simulink model "Model_14Bus_Microgrid_paper_Latam"  (R2022b)
settings: Solver=VariableStepAuto  StartTime=0.0  StopTime=0.5  MaxStep=1e-2  RelTol=1e-3
InitFcn:
  | Set_parameters_R2018
StopFcn:
  | %Save_Data;
  | %Graphics_mod;
values from neighbouring files (symbols this model uses):
  Clink = Ceq*2    (= 0.217013888889)    [Set_parameters.m]
  dis1 = 0.15    [Set_parameters.m]
  dis10 = 6    [Set_parameters.m]
  dis11 = 3    [Set_parameters.m]
  dis12 = 6    [Set_parameters.m]
  dis13 = 3    [Set_parameters.m]
  dis14 = 2    [Set_parameters.m]
  dis2 = 0.2    [Set_parameters.m]
  dis3 = 0.15    [Set_parameters.m]
  dis4 = 0.4    [Set_parameters.m]
  dis5 = 0.4    [Set_parameters.m]
  dis6 = 0.4    [Set_parameters.m]
  dis7 = 0.1    [Set_parameters.m]
  dis8 = 2    [Set_parameters.m]
  dis9 = 6    [Set_parameters.m]
  Fc = 33 * Fnom    (= 1980)    [Set_parameters.m]
  Fnom = 60    [Set_parameters.m]
  Increment_MPPT = 0.01    [Set_parameters.m]
  Ki_Ireg = 20    [Set_parameters.m]
  Ki_VDCreg = 400    [Set_parameters.m]
  Kp_Ireg = 0.3    [Set_parameters.m]
  Kp_VDCreg = 2    [Set_parameters.m]
  LimitL_Ireg = -1.5    [Set_parameters.m]
  LimitL_VDCreg = -1.5    [Set_parameters.m]
  Limits_MPPT = [ 583 357 ]    [Set_parameters.m]
  LimitU_Ireg = 1.5    [Set_parameters.m]
  LimitU_VDCreg = 1.5    [Set_parameters.m]
  P_Load_2 = S_Load_2* PF_Load_2    (= 36000)    [Set_parameters.m]
  P_Load_3 = S_Load_3* PF_Load_3    (= 25500)    [Set_parameters.m]
  Pnom = 1e6    (= 1000000)    [Set_parameters.m]
  Pnom_T1 = 1.5e6    (= 1500000)    [Set_parameters.m]
  Pnom_T2 = 1.5e6    (= 1500000)    [Set_parameters.m]
  Pnom_T3 = 4e6    (= 4000000)    [Set_parameters.m]
  Pnom_xfo = Pnom    (= 1000000)    [Set_parameters.m]
  Ql_Load_2 = S_Load_2 * sin(acos(PF_Load_2))    [Set_parameters.m]
  Ql_Load_3 = S_Load_3 * sin(acos(PF_Load_3))    [Set_parameters.m]
  R_Load_9 = (Vnom_prim * 1.35)^2 / P_Load_9    (= 1084.6153125)    [Set_parameters.m]
  R_Load_DC = Vnom_DC^2/ P_Load_DC    (= 45)    [Set_parameters.m]
  Rl = 0.394    [Set_parameters.m]
  Rls = 0.198    [Set_parameters.m]
  Ts = Ts_Power    (= 5.05050505051e-06)    [Set_parameters.m]
  Ts_Control = 10*Ts_Power    (= 5.05050505051e-05)    [Set_parameters.m]
  Ts_Power = 1/(33*Fnom)/100    (= 5.05050505051e-06)    [Set_parameters.m]
  V1_LL_T3 = 69e3    (= 69000)    [Set_parameters.m]
  Vf = 0    [Set_parameters.m]
  Vfd = 0    [Set_parameters.m]
  Vnom_dc = 480    [Set_parameters.m]
  Vnom_Diesel = 2.4e3    (= 2400)    [Set_parameters.m]
  Vnom_prim = 13.8e3    (= 13800)    [Set_parameters.m]
  Vnom_sec = 220    [Set_parameters.m]
  Vnom_ter_AC_DC = 150    [Set_parameters.m]
  Xl = 0.1168    [Set_parameters.m]
  Xls = 0.1089    [Set_parameters.m]
undefined symbols (not defined in the file or in its folder): D1, Delta, DiscIntNeverNeededParam, Hydride, Ion, level, Lithium, max_min, Metal, Nickel, RL, RLff, sigbuilder_block
libraries: spsRMSLib x73, powerlib_extras x53, spsCurrentMeasurementLib x47, spsTHDLib x26, spsThreePhaseVIMeasurementLib x25, spsVoltageMeasurementLib x23, spsSeriesRLCBranchLib x21, spsThreePhaseSeriesRLCBranchLib x21, spsIGBTDiodeLib x15, spsThreePhaseBreakerLib x14, spsPowerLib x14, spsThreePhaseTransformerTwoWindingsLib x12
(part 2 of 10)

== system Model_14Bus_Microgrid_paper_Latam/BESS ==
  note: B1 + -
  note: + - B3
  note: + - B2
  note: DC Bus
  note: AC Bus
  note: ---------------
  note: -----------------
  "BESS " : Subsystem
      mask Display: image('/Users/christian/Documents/MATLAB/doctorado/4 conectada a la red con generador diesel, con generacion renovanble (fv)-con almacenamiento varios scope/Icons/Battery Energy Storage System (BESS).png'); % Use "Edit Image" on toolstrip to change.
  "Breaker BESS " : spsThreePhaseBreakerLib/Three-Phase Breaker  InitialState=closed  SwitchA=on  SwitchB=on  SwitchC=on  SwitchTimes="[4/60  10/60]"  External=on  BreakerResistance=0.001  SnubberResistance=1e6  SnubberCapacitance=inf  Measurements=None
  On/off Bess : Constant
  TB 900 V / 220 V 55 kVA : spsThreePhaseTransformerTwoWindingsLib/Three-Phase Transformer (Two Windings)  Winding1Connection=Delta (D1)  Winding2Connection=Y  CoreType=Three single-phase transformers  SetSaturation=off  Hysteresis=off  DataFile='hysteresis'  SetInitialFlux=off  Measurements=None  UNITS=pu  NominalPower=[ 55e3 , Fnom ]  Winding1=[ 900 , 0.0015 , 0.03]  Winding2=[ Vnom_sec , 0.0015 , 0.03 ]  Rm=200  Lm=200  L0=0.5  Saturation="[ 0,0  ;  0.005,1.2  ;  1.0,1.4 ]"  InitialFluxes=[ 0.8 , -0.8 , 0.7 ]  BreakLoop=off  DiscreteSolver=Trapezoidal iterative  DataType=off  TransfoNumber=0
  convertidor bidireccional AC/DC : Subsystem
      mask Display: image('/Users/christian/Documents/MATLAB/doctorado/4 conectada a la red con generador diesel, con generacion renovanble (fv)-con almacenamiento varios scope/Icons/Bi-directional converter.png'); % Use "Edit Image" on toolstrip to change.
  a : PMIOPort  Side=Right
  b : PMIOPort  Port=2  Side=Right
  c : PMIOPort  Port=3  Side=Right
  wires:
  On/off Bess/1 -> "Breaker BESS "/1
  connections:
  a/RConn1 -- "Breaker BESS "/RConn1
  TB 900 V / 220 V 55 kVA/LConn1 -- convertidor bidireccional AC/DC/LConn3
  TB 900 V / 220 V 55 kVA/RConn3 -- "Breaker BESS "/LConn3
  "BESS "/LConn5 -- convertidor bidireccional AC/DC/RConn2
  "Breaker BESS "/RConn3 -- c/RConn1
  "BESS "/LConn6 -- convertidor bidireccional AC/DC/RConn1
  TB 900 V / 220 V 55 kVA/LConn2 -- convertidor bidireccional AC/DC/LConn2
  TB 900 V / 220 V 55 kVA/LConn3 -- convertidor bidireccional AC/DC/LConn1
  "BESS "/LConn2 -- convertidor bidireccional AC/DC/RConn5
  "BESS "/LConn4 -- convertidor bidireccional AC/DC/RConn3
  TB 900 V / 220 V 55 kVA/RConn2 -- "Breaker BESS "/LConn2
  b/RConn1 -- "Breaker BESS "/RConn2
  TB 900 V / 220 V 55 kVA/RConn1 -- "Breaker BESS "/LConn1
  "BESS "/LConn1 -- convertidor bidireccional AC/DC/RConn6
  "BESS "/LConn3 -- convertidor bidireccional AC/DC/RConn4

== system Model_14Bus_Microgrid_paper_Latam/BESS2 ==
  note: ---------------------------------------------------------------------------
  Breaker : spsBreakerLib/Breaker  InitialState=1  SwitchingTimes="[1/60  5/60]"  External=on  BreakerResistance=0.01  SnubberResistance=1e6  SnubberCapacitance=inf  Measurements=None  MoreParameters=on  NoBreakLoop=off
  Breaker1 : spsBreakerLib/Breaker  InitialState=1  SwitchingTimes="[1/60  5/60]"  External=on  BreakerResistance=0.01  SnubberResistance=1e6  SnubberCapacitance=inf  Measurements=None  MoreParameters=on  NoBreakLoop=off
  Current Measurement1 : spsCurrentMeasurementLib/Current Measurement  PhasorSimulation=off  OutputType=Complex  PSBequivalent=0
  On/off 1 : Constant
  Subsystem2 : Subsystem
  1 : PMIOPort  Side=Left
  2 : PMIOPort  Port=2  Side=Left
  3 : PMIOPort  Port=3  Side=Right
  4 : PMIOPort  Port=4  Side=Right
  tag scope: I_BusDC=global
  wires:
  Current Measurement1/1 -> [I_BusDC]
  On/off 1/1 -> Breaker1/1, Breaker/1
  connections:
  1/RConn1 -- Breaker1/RConn1
  2/RConn1 -- Breaker/RConn1
  Subsystem2/RConn2 -- Breaker1/LConn1 -- 3/RConn1
  Current Measurement1/LConn1 -- Subsystem2/RConn1 -- 4/RConn1
  Current Measurement1/RConn1 -- Breaker/LConn1

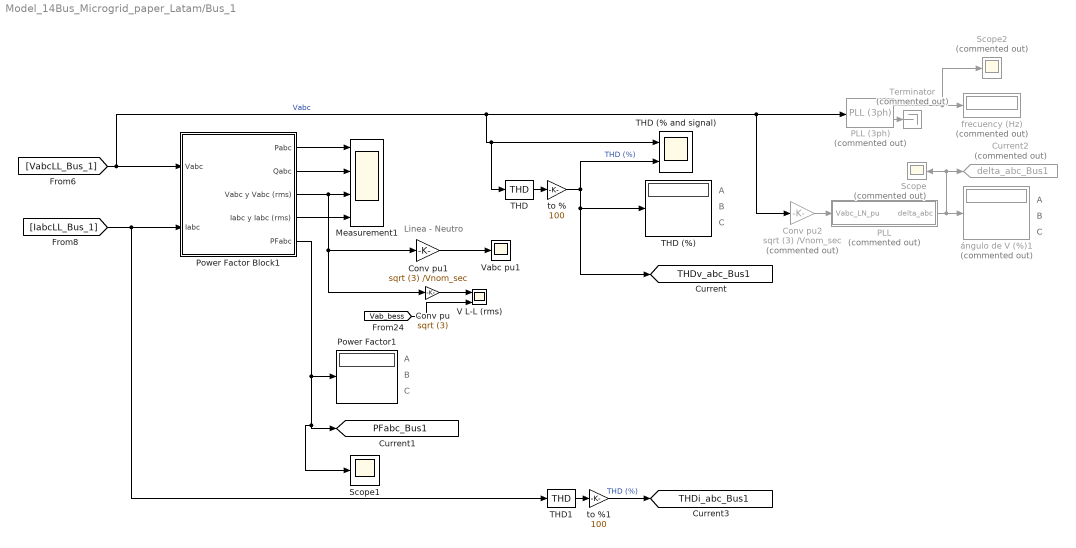
== system Model_14Bus_Microgrid_paper_Latam/Bus_1 ==
  note: C
  note: B
  note: A
  note: C
  note: Linea - Neutro
  note: B
  note: A
  note: A
  note: C
  note: B
  Conv pu : Gain  Gain=sqrt (3)  SaturateOnIntegerOverflow=on  OutDataTypeStr=Inherit: Same as input  ParamDataTypeStr=Inherit: Same as input
  Conv pu1 : Gain  Gain=sqrt (3) /Vnom_sec  SaturateOnIntegerOverflow=on  OutDataTypeStr=Inherit: Same as input  ParamDataTypeStr=Inherit: Same as input
  Conv pu2 : Gain  Commented=on  Gain=sqrt (3) /Vnom_sec  SaturateOnIntegerOverflow=on  OutDataTypeStr=Inherit: Same as input  ParamDataTypeStr=Inherit: Same as input
  Current2 : Goto  Commented=on  GotoTag=delta_abc_Bus1  TagVisibility=global
  Measurement1 : Scope  NumInputPorts=4
  PLL : Subsystem  Commented=on
  PLL (3ph) : spsPLL3phLib/PLL (3ph)  Commented=on  Fmin=45  Par_Init=[0, 60]  ParK=[180, 3200, 1]  TcD=1e-4  MaxRateChangeFreq=12  FilterCutOffFreq=25  Ts=0  AGC=on
  Power Factor Block1 : Subsystem  mask(Power Factor Block){Freq=Fnom, Vinit=[0, 0], Iinit=[0, 0], Ts=0}
      mask prompts: Freq "Fundamental frequency (Hz):"; Vinit "Voltage initial input [ Mag, Phase (degrees) ]:"; Iinit "Current initial input [ Mag, Phase (degrees) ]:"; Ts "Sample time:"
      mask help:
      | Power Factor Block developed by Dr Rodney Tan
      | Version 1.01 (Aug 2016)
      |
      | Compute power factor and phase angle of AC circuit voltage-current pair at fundamental frequency.
      |
      | The computation is based on Power block and Complex number function block.
      |
      | For the first cycle of simulation, the outputs are held constant to the powers computed for the Voltage initial input and Current initial input parameters.
      mask Help:
      | <b>Fundamental Frequency (Hz)</b>
      | Specify the measurement fundamental frequency, in hertz, of the input signal.
      | 
      | <b>Voltage initial input [ Mag, Phase (degrees) ]</b>
      | Specify the voltage initial magnitude and phase to set a constant output for the first cycle of simulation.
      | 
      | <b>Current initial input [ Mag, Phase (degrees) ]</b>
      | Specify the current initial magnitude and phase to set a constant output for the first cycle of simulation.
      | 
      | <b>Sample Time</b>
      | Specify the sample time of the block, in seconds. Set to 0 to implement a continuous block.
      mask TypeOptions Freq: Power/Freq
      mask TypeOptions Vinit: Power/Vinit
      mask TypeOptions Iinit: Power/Iinit
      mask TypeOptions Ts: Power/Ts
  Power Factor1 : Display
  Scope : Scope  Commented=on
  Scope1 : Scope
  Scope2 : Scope  Commented=on
  THD : spsTHDLib/THD  Freq=60  Ts=Ts_Power
  THD (% and signal) : Scope  NumInputPorts=2
  THD (%) : Display
      settings: Format=bank
  THD1 : spsTHDLib/THD  Freq=60  Ts=Ts_Power
  Terminator : Terminator  Commented=on
  V L-L (rms) : Scope  NumInputPorts=2
  Vabc pu1 : Scope
  frecuency (Hz) : Display  Commented=on
  to % : Gain  Gain=100  SampleTime=Ts_Power
  to %1 : Gain  Gain=100  SampleTime=Ts_Power
  ángulo de V (%)1 : Display  Commented=on
      settings: Format=bank
  tag scope: PFabc_Bus1=global, THDi_abc_Bus1=global, THDv_abc_Bus1=global
  wires:
  THD/1 -> to %/1
  to %/1 -> [THDv_abc_Bus1], THD (%)/1, THD (% and signal)/2  "THD (%)"
  Power Factor Block1/4(Iabc y Iabc (rms)) -> Measurement1/4
  Power Factor Block1/1(Pabc) -> Measurement1/1
  Conv pu1/1 -> Vabc pu1/1
  Power Factor Block1/5("PFabc ") -> Power Factor1/1, Scope1/1, [PFabc_Bus1]
  Power Factor Block1/2(Qabc) -> Measurement1/2
  Power Factor Block1/3(Vabc y Vabc (rms)) -> Conv pu/1, Conv pu1/1, Measurement1/3
  [IabcLL_Bus_1] -> THD1/1, Power Factor Block1/2(Iabc)
  Conv pu/1 -> V L-L (rms)/1
  [Vab_bess] -> V L-L (rms)/2
  PLL/1(delta_abc) -> Current2/1, Scope/1, ángulo de V (%)1/1
  Conv pu2/1 -> PLL/1(Vabc_LN_pu)
  PLL (3ph)/2 -> Terminator/1
  [VabcLL_Bus_1] -> Power Factor Block1/1(Vabc), PLL (3ph)/1, Conv pu2/1, THD/1, THD (% and signal)/1  "Vabc"
  PLL (3ph)/1 -> Scope2/1, frecuency (Hz)/1
  THD1/1 -> to %1/1
  to %1/1 -> [THDi_abc_Bus1]  "THD (%)"

== system Model_14Bus_Microgrid_paper_Latam/Bus_14  ==
  note: C
  note: B
  note: A
  note: C
  note: Linea - Neutro
  note: B
  note: A
  note: A
  note: B
  Conv pu1 : Gain  Gain=sqrt (3) /Vnom_prim  SaturateOnIntegerOverflow=on  OutDataTypeStr=Inherit: Same as input  ParamDataTypeStr=Inherit: Same as input
  Conv pu2 : Gain  Commented=on  Gain=sqrt (3) /Vnom_prim  SaturateOnIntegerOverflow=on  OutDataTypeStr=Inherit: Same as input  ParamDataTypeStr=Inherit: Same as input
  Current2 : Goto  Commented=on  GotoTag=delta_abc_Bus14  TagVisibility=global
  Gain : Gain  Gain=-1
  Measurement1 : Scope  NumInputPorts=4
  PLL : Subsystem  Commented=on
  Power Factor Block1 : Subsystem  mask(Power Factor Block){Freq=Fnom, Vinit=[0, 0], Iinit=[0, 0], Ts=0}
      mask prompts: Freq "Fundamental frequency (Hz):"; Vinit "Voltage initial input [ Mag, Phase (degrees) ]:"; Iinit "Current initial input [ Mag, Phase (degrees) ]:"; Ts "Sample time:"
      mask help:
      | Power Factor Block developed by Dr Rodney Tan
      | Version 1.01 (Aug 2016)
      |
      | Compute power factor and phase angle of AC circuit voltage-current pair at fundamental frequency.
      |
      | The computation is based on Power block and Complex number function block.
      |
      | For the first cycle of simulation, the outputs are held constant to the powers computed for the Voltage initial input and Current initial input parameters.
      mask Help:
      | <b>Fundamental Frequency (Hz)</b>
      | Specify the measurement fundamental frequency, in hertz, of the input signal.
      | 
      | <b>Voltage initial input [ Mag, Phase (degrees) ]</b>
      | Specify the voltage initial magnitude and phase to set a constant output for the first cycle of simulation.
      | 
      | <b>Current initial input [ Mag, Phase (degrees) ]</b>
      | Specify the current initial magnitude and phase to set a constant output for the first cycle of simulation.
      | 
      | <b>Sample Time</b>
      | Specify the sample time of the block, in seconds. Set to 0 to implement a continuous block.
      mask TypeOptions Freq: Power/Freq
      mask TypeOptions Vinit: Power/Vinit
      mask TypeOptions Iinit: Power/Iinit
      mask TypeOptions Ts: Power/Ts
  Power Factor1 : Display
  Scope : Scope  Commented=on
  THD : spsTHDLib/THD  Freq=60  Ts=Ts_Power
  THD (% and signal) : Scope  NumInputPorts=2
  THD (%) : Display
      settings: Format=bank
  THD1 : spsTHDLib/THD  Freq=60  Ts=Ts_Power
  Vabc pu1 : Scope
  to % : Gain  Gain=100  SampleTime=Ts_Power
  to %1 : Gain  Gain=100  SampleTime=Ts_Power
  ángulo de V (%)1 : Display  Commented=on
      settings: Format=bank
  tag scope: PFabc_Bus14=global, THDi_abc_Bus14=global, THDv_abc_Bus14=global
  wires:
  [IabcLL_Bus_14] -> THD1/1, Power Factor Block1/2(Iabc)
  THD/1 -> to %/1
  Power Factor Block1/4(Iabc y Iabc (rms)) -> Measurement1/4
  Power Factor Block1/1(Pabc) -> Measurement1/1
  Conv pu1/1 -> Vabc pu1/1
  Power Factor Block1/2(Qabc) -> Measurement1/2
  Power Factor Block1/3(Vabc y Vabc (rms)) -> Conv pu1/1, Measurement1/3
  to %/1 -> [THDv_abc_Bus14], THD (%)/1, THD (% and signal)/2  "THD (%)"
  Power Factor Block1/5("PFabc ") -> Gain/1
  PLL/1(delta_abc) -> Current2/1, Scope/1, ángulo de V (%)1/1
  [VabcLL_Bus_14] -> Power Factor Block1/1(Vabc), Conv pu2/1, THD/1, THD (% and signal)/1  "Signal Vabc"
  Conv pu2/1 -> PLL/1(Vabc_LN_pu)
  Gain/1 -> [PFabc_Bus14], Power Factor1/1
  THD1/1 -> to %1/1
  to %1/1 -> [THDi_abc_Bus14]  "THD (%)"

== system Model_14Bus_Microgrid_paper_Latam/Bus_2 ==
  note: C
  note: B
  note: A
  note: A
  note: B
  note: Linea - Neutro
  note: C
  note: A
  note: B
  note: C
  Conv pu1 : Gain  Gain=sqrt (3) /Vnom_sec  SaturateOnIntegerOverflow=on  OutDataTypeStr=Inherit: Same as input  ParamDataTypeStr=Inherit: Same as input
  Conv pu2 : Gain  Commented=on  Gain=sqrt (3) /Vnom_sec  SaturateOnIntegerOverflow=on  OutDataTypeStr=Inherit: Same as input  ParamDataTypeStr=Inherit: Same as input
  Current2 : Goto  Commented=on  GotoTag=delta_abc_Bus2  TagVisibility=global
  Measurement1 : Scope  NumInputPorts=4
  PLL : Subsystem  Commented=on
  PLL (3ph) : spsPLL3phLib/PLL (3ph)  Commented=on  Fmin=45  Par_Init=[0, 60]  ParK=[180, 3200, 1]  TcD=1e-4  MaxRateChangeFreq=12  FilterCutOffFreq=25  Ts=0  AGC=on
  Power Factor Block1 : Subsystem  mask(Power Factor Block){Freq=Fnom, Vinit=[0, 0], Iinit=[0, 0], Ts=0}
      mask prompts: Freq "Fundamental frequency (Hz):"; Vinit "Voltage initial input [ Mag, Phase (degrees) ]:"; Iinit "Current initial input [ Mag, Phase (degrees) ]:"; Ts "Sample time:"
      mask help:
      | Power Factor Block developed by Dr Rodney Tan
      | Version 1.01 (Aug 2016)
      |
      | Compute power factor and phase angle of AC circuit voltage-current pair at fundamental frequency.
      |
      | The computation is based on Power block and Complex number function block.
      |
      | For the first cycle of simulation, the outputs are held constant to the powers computed for the Voltage initial input and Current initial input parameters.
      mask Help:
      | <b>Fundamental Frequency (Hz)</b>
      | Specify the measurement fundamental frequency, in hertz, of the input signal.
      | 
      | <b>Voltage initial input [ Mag, Phase (degrees) ]</b>
      | Specify the voltage initial magnitude and phase to set a constant output for the first cycle of simulation.
      | 
      | <b>Current initial input [ Mag, Phase (degrees) ]</b>
      | Specify the current initial magnitude and phase to set a constant output for the first cycle of simulation.
      | 
      | <b>Sample Time</b>
      | Specify the sample time of the block, in seconds. Set to 0 to implement a continuous block.
      mask TypeOptions Freq: Power/Freq
      mask TypeOptions Vinit: Power/Vinit
      mask TypeOptions Iinit: Power/Iinit
      mask TypeOptions Ts: Power/Ts
  Power Factor1 : Display
  Scope : Scope  Commented=on
  Scope2 : Scope  Commented=on
  THD : spsTHDLib/THD  Freq=60  Ts=Ts_Power
  THD (% and signal) : Scope  NumInputPorts=2
  THD (%) : Display
      settings: Format=bank
  THD1 : spsTHDLib/THD  Freq=60  Ts=Ts_Power
  Terminator : Terminator  Commented=on
  Vabc pu1 : Scope
  frecuency (Hz) : Display  Commented=on
  to % : Gain  Gain=100  SampleTime=Ts_Power
  to %1 : Gain  Gain=100  SampleTime=Ts_Power
  ángulo de V (%)1 : Display  Commented=on
      settings: Format=bank
  tag scope: PFabc_Bus2=global, THDi_abc_Bus2=global, THDv_abc_Bus2=global
  wires:
  [IabcLL_Bus_2] -> THD1/1, Power Factor Block1/2(Iabc)
  THD/1 -> to %/1
  Power Factor Block1/3(Vabc y Vabc (rms)) -> Conv pu1/1, Measurement1/3
  Power Factor Block1/4(Iabc y Iabc (rms)) -> Measurement1/4
  Conv pu1/1 -> Vabc pu1/1
  Power Factor Block1/2(Qabc) -> Measurement1/2
  Power Factor Block1/1(Pabc) -> Measurement1/1
  Power Factor Block1/5("PFabc ") -> [PFabc_Bus2], Power Factor1/1
  to %/1 -> [THDv_abc_Bus2], THD (%)/1, THD (% and signal)/2  "THD (%)"
  Conv pu2/1 -> PLL/1(Vabc_LN_pu)
  PLL/1(delta_abc) -> Current2/1, Scope/1, ángulo de V (%)1/1
  PLL (3ph)/2 -> Terminator/1
  [VabcLL_Bus_2] -> PLL (3ph)/1, Conv pu2/1, THD/1, THD (% and signal)/1, Power Factor Block1/1(Vabc)  "Vabc"
  PLL (3ph)/1 -> Scope2/1, frecuency (Hz)/1
  THD1/1 -> to %1/1
  to %1/1 -> [THDi_abc_Bus2]  "THD (%)"

== system Model_14Bus_Microgrid_paper_Latam/Bus_3 ==
  note: C
  note: B
  note: A
  note: C
  note: Linea - Neutro
  note: B
  note: A
  note: A
  note: B
  note: C
  Conv pu1 : Gain  Gain=sqrt (3) /Vnom_sec  SaturateOnIntegerOverflow=on  OutDataTypeStr=Inherit: Same as input  ParamDataTypeStr=Inherit: Same as input
  Conv pu2 : Gain  Commented=on  Gain=sqrt (3) /Vnom_sec  SaturateOnIntegerOverflow=on  OutDataTypeStr=Inherit: Same as input  ParamDataTypeStr=Inherit: Same as input
  Current2 : Goto  Commented=on  GotoTag=delta_abc_Bus3  TagVisibility=global
  Measurement1 : Scope  NumInputPorts=4
  PLL : Subsystem  Commented=on
  Power Factor Block1 : Subsystem  mask(Power Factor Block){Freq=Fnom, Vinit=[0, 0], Iinit=[0, 0], Ts=0}
      mask prompts: Freq "Fundamental frequency (Hz):"; Vinit "Voltage initial input [ Mag, Phase (degrees) ]:"; Iinit "Current initial input [ Mag, Phase (degrees) ]:"; Ts "Sample time:"
      mask help:
      | Power Factor Block developed by Dr Rodney Tan
      | Version 1.01 (Aug 2016)
      |
      | Compute power factor and phase angle of AC circuit voltage-current pair at fundamental frequency.
      |
      | The computation is based on Power block and Complex number function block.
      |
      | For the first cycle of simulation, the outputs are held constant to the powers computed for the Voltage initial input and Current initial input parameters.
      mask Help:
      | <b>Fundamental Frequency (Hz)</b>
      | Specify the measurement fundamental frequency, in hertz, of the input signal.
      | 
      | <b>Voltage initial input [ Mag, Phase (degrees) ]</b>
      | Specify the voltage initial magnitude and phase to set a constant output for the first cycle of simulation.
      | 
      | <b>Current initial input [ Mag, Phase (degrees) ]</b>
      | Specify the current initial magnitude and phase to set a constant output for the first cycle of simulation.
      | 
      | <b>Sample Time</b>
      | Specify the sample time of the block, in seconds. Set to 0 to implement a continuous block.
      mask TypeOptions Freq: Power/Freq
      mask TypeOptions Vinit: Power/Vinit
      mask TypeOptions Iinit: Power/Iinit
      mask TypeOptions Ts: Power/Ts
  Power Factor1 : Display
  Scope : Scope  Commented=on
  THD : spsTHDLib/THD  Freq=60  Ts=Ts_Power
  THD (% and signal) : Scope  NumInputPorts=2
  THD (%) : Display
      settings: Format=bank
  THD1 : spsTHDLib/THD  Freq=60  Ts=Ts_Power
  Vabc pu1 : Scope
  to % : Gain  Gain=100  SampleTime=Ts_Power
  to %1 : Gain  Gain=100  SampleTime=Ts_Power
  ángulo de V (%)1 : Display  Commented=on
      settings: Format=bank
  tag scope: PFabc_Bus3=global, THDi_abc_Bus3=global, THDv_abc_Bus3=global
  wires:
  [IabcLL_Bus_3] -> THD1/1, Power Factor Block1/2(Iabc)
  THD/1 -> to %/1
  Power Factor Block1/4(Iabc y Iabc (rms)) -> Measurement1/4
  Power Factor Block1/1(Pabc) -> Measurement1/1
  Conv pu1/1 -> Vabc pu1/1
  Power Factor Block1/2(Qabc) -> Measurement1/2
  Power Factor Block1/3(Vabc y Vabc (rms)) -> Conv pu1/1, Measurement1/3
  Power Factor Block1/5("PFabc ") -> [PFabc_Bus3], Power Factor1/1
  to %/1 -> [THDv_abc_Bus3], THD (%)/1, THD (% and signal)/2  "THD (%)"
  Conv pu2/1 -> PLL/1(Vabc_LN_pu)
  PLL/1(delta_abc) -> Current2/1, Scope/1, ángulo de V (%)1/1
  [VabcLL_Bus_3] -> Conv pu2/1, THD/1, THD (% and signal)/1, Power Factor Block1/1(Vabc)  "Signal Vabc"
  THD1/1 -> to %1/1
  to %1/1 -> [THDi_abc_Bus3]  "THD (%)"

== system Model_14Bus_Microgrid_paper_Latam/Bus_4 ==
  note: C
  note: B
  note: A
  note: C
  note: Linea - Neutro
  note: B
  note: A
  note: A
  note: B
  note: C
  Conv pu1 : Gain  Gain=sqrt (3) /Vnom_sec  SaturateOnIntegerOverflow=on  OutDataTypeStr=Inherit: Same as input  ParamDataTypeStr=Inherit: Same as input
  Conv pu2 : Gain  Commented=on  Gain=sqrt (3) /Vnom_sec  SaturateOnIntegerOverflow=on  OutDataTypeStr=Inherit: Same as input  ParamDataTypeStr=Inherit: Same as input
  Current2 : Goto  Commented=on  GotoTag=delta_abc_Bus4  TagVisibility=global
  Measurement1 : Scope  NumInputPorts=4
  PLL : Subsystem  Commented=on
  Power Factor Block1 : Subsystem  mask(Power Factor Block){Freq=Fnom, Vinit=[0, 0], Iinit=[0, 0], Ts=0}
      mask prompts: Freq "Fundamental frequency (Hz):"; Vinit "Voltage initial input [ Mag, Phase (degrees) ]:"; Iinit "Current initial input [ Mag, Phase (degrees) ]:"; Ts "Sample time:"
      mask help:
      | Power Factor Block developed by Dr Rodney Tan
      | Version 1.01 (Aug 2016)
      |
      | Compute power factor and phase angle of AC circuit voltage-current pair at fundamental frequency.
      |
      | The computation is based on Power block and Complex number function block.
      |
      | For the first cycle of simulation, the outputs are held constant to the powers computed for the Voltage initial input and Current initial input parameters.
      mask Help:
      | <b>Fundamental Frequency (Hz)</b>
      | Specify the measurement fundamental frequency, in hertz, of the input signal.
      | 
      | <b>Voltage initial input [ Mag, Phase (degrees) ]</b>
      | Specify the voltage initial magnitude and phase to set a constant output for the first cycle of simulation.
      | 
      | <b>Current initial input [ Mag, Phase (degrees) ]</b>
      | Specify the current initial magnitude and phase to set a constant output for the first cycle of simulation.
      | 
      | <b>Sample Time</b>
      | Specify the sample time of the block, in seconds. Set to 0 to implement a continuous block.
      mask TypeOptions Freq: Power/Freq
      mask TypeOptions Vinit: Power/Vinit
      mask TypeOptions Iinit: Power/Iinit
      mask TypeOptions Ts: Power/Ts
  Power Factor1 : Display
  Scope : Scope  Commented=on
  THD : spsTHDLib/THD  Freq=60  Ts=Ts_Power
  THD (% and signal) : Scope  NumInputPorts=2
  THD (%) : Display
      settings: Format=bank
  THD1 : spsTHDLib/THD  Freq=60  Ts=Ts_Power
  Vabc pu1 : Scope
  to % : Gain  Gain=100  SampleTime=Ts_Power
  to %1 : Gain  Gain=100  SampleTime=Ts_Power
  ángulo de V (%)1 : Display  Commented=on
      settings: Format=bank
  tag scope: PFabc_Bus4=global, THDi_abc_Bus4=global, THDv_abc_Bus4=global
  wires:
  [IabcLL_Bus_4] -> THD1/1, Power Factor Block1/2(Iabc)
  THD/1 -> to %/1
  Power Factor Block1/4(Iabc y Iabc (rms)) -> Measurement1/4
  Power Factor Block1/1(Pabc) -> Measurement1/1
  Conv pu1/1 -> Vabc pu1/1
  Power Factor Block1/2(Qabc) -> Measurement1/2
  Power Factor Block1/3(Vabc y Vabc (rms)) -> Conv pu1/1, Measurement1/3
  Power Factor Block1/5("PFabc ") -> [PFabc_Bus4], Power Factor1/1
  to %/1 -> [THDv_abc_Bus4], THD (%)/1, THD (% and signal)/2  "THD (%)"
  Conv pu2/1 -> PLL/1(Vabc_LN_pu)
  PLL/1(delta_abc) -> Current2/1, Scope/1, ángulo de V (%)1/1
  [VabcLL_Bus_4] -> Power Factor Block1/1(Vabc), Conv pu2/1, THD/1, THD (% and signal)/1  "Signal Vabc"
  THD1/1 -> to %1/1
  to %1/1 -> [THDi_abc_Bus4]  "THD (%)"

== system Model_14Bus_Microgrid_paper_Latam/Bus_5 ==
  note: C
  note: B
  note: A
  note: C
  note: Linea - Neutro
  note: B
  note: A
  note: A
  note: B
  note: C
  Conv pu1 : Gain  Gain=sqrt (3) /Vnom_sec  SaturateOnIntegerOverflow=on  OutDataTypeStr=Inherit: Same as input  ParamDataTypeStr=Inherit: Same as input
  Conv pu2 : Gain  Commented=on  Gain=sqrt (3) /Vnom_sec  SaturateOnIntegerOverflow=on  OutDataTypeStr=Inherit: Same as input  ParamDataTypeStr=Inherit: Same as input
  Current2 : Goto  Commented=on  GotoTag=delta_abc_Bus5  TagVisibility=global
  Measurement1 : Scope  NumInputPorts=4
  PLL : Subsystem  Commented=on
  Power Factor Block1 : Subsystem  mask(Power Factor Block){Freq=Fnom, Vinit=[0, 0], Iinit=[0, 0], Ts=0}
      mask prompts: Freq "Fundamental frequency (Hz):"; Vinit "Voltage initial input [ Mag, Phase (degrees) ]:"; Iinit "Current initial input [ Mag, Phase (degrees) ]:"; Ts "Sample time:"
      mask help:
      | Power Factor Block developed by Dr Rodney Tan
      | Version 1.01 (Aug 2016)
      |
      | Compute power factor and phase angle of AC circuit voltage-current pair at fundamental frequency.
      |
      | The computation is based on Power block and Complex number function block.
      |
      | For the first cycle of simulation, the outputs are held constant to the powers computed for the Voltage initial input and Current initial input parameters.
      mask Help:
      | <b>Fundamental Frequency (Hz)</b>
      | Specify the measurement fundamental frequency, in hertz, of the input signal.
      | 
      | <b>Voltage initial input [ Mag, Phase (degrees) ]</b>
      | Specify the voltage initial magnitude and phase to set a constant output for the first cycle of simulation.
      | 
      | <b>Current initial input [ Mag, Phase (degrees) ]</b>
      | Specify the current initial magnitude and phase to set a constant output for the first cycle of simulation.
      | 
      | <b>Sample Time</b>
      | Specify the sample time of the block, in seconds. Set to 0 to implement a continuous block.
      mask TypeOptions Freq: Power/Freq
      mask TypeOptions Vinit: Power/Vinit
      mask TypeOptions Iinit: Power/Iinit
      mask TypeOptions Ts: Power/Ts
  Power Factor1 : Display
  Scope : Scope  Commented=on
  THD : spsTHDLib/THD  Freq=60  Ts=Ts_Power
  THD (% and signal) : Scope  NumInputPorts=2
  THD (%) : Display
      settings: Format=bank
  THD1 : spsTHDLib/THD  Freq=60  Ts=Ts_Power
  Vabc pu1 : Scope
  to % : Gain  Gain=100  SampleTime=Ts_Power
  to %1 : Gain  Gain=100  SampleTime=Ts_Power
  ángulo de V (%)1 : Display  Commented=on
      settings: Format=bank
  tag scope: PFabc_Bus5=global, THDi_abc_Bus5=global, THDv_abc_Bus5=global
  wires:
  [IabcLL_Bus_5] -> THD1/1, Power Factor Block1/2(Iabc)
  THD/1 -> to %/1
  Power Factor Block1/4(Iabc y Iabc (rms)) -> Measurement1/4
  Power Factor Block1/1(Pabc) -> Measurement1/1
  Conv pu1/1 -> Vabc pu1/1
  Power Factor Block1/2(Qabc) -> Measurement1/2
  Power Factor Block1/3(Vabc y Vabc (rms)) -> Conv pu1/1, Measurement1/3
  Power Factor Block1/5("PFabc ") -> [PFabc_Bus5], Power Factor1/1
  to %/1 -> [THDv_abc_Bus5], THD (%)/1, THD (% and signal)/2  "THD (%)"
  Conv pu2/1 -> PLL/1(Vabc_LN_pu)
  PLL/1(delta_abc) -> Current2/1, Scope/1, ángulo de V (%)1/1
  [VabcLL_Bus_5] -> Power Factor Block1/1(Vabc), Conv pu2/1, THD/1, THD (% and signal)/1  "Signal Vabc"
  THD1/1 -> to %1/1
  to %1/1 -> [THDi_abc_Bus5]  "THD (%)"

== system Model_14Bus_Microgrid_paper_Latam/Bus_6 ==
  note: C
  note: B
  note: A
  note: C
  note: Linea - Neutro
  note: B
  note: A
  note: A
  note: B
  note: C
  Conv pu1 : Gain  Gain=sqrt (3) /Vnom_sec  SaturateOnIntegerOverflow=on  OutDataTypeStr=Inherit: Same as input  ParamDataTypeStr=Inherit: Same as input
  Conv pu2 : Gain  Commented=on  Gain=sqrt (3) /Vnom_sec  SaturateOnIntegerOverflow=on  OutDataTypeStr=Inherit: Same as input  ParamDataTypeStr=Inherit: Same as input
  Current2 : Goto  Commented=on  GotoTag=delta_abc_Bus4  TagVisibility=global
  Measurement1 : Scope  NumInputPorts=4
  PLL : Subsystem  Commented=on
  Power Factor Block1 : Subsystem  mask(Power Factor Block){Freq=Fnom, Vinit=[0, 0], Iinit=[0, 0], Ts=0}
      mask prompts: Freq "Fundamental frequency (Hz):"; Vinit "Voltage initial input [ Mag, Phase (degrees) ]:"; Iinit "Current initial input [ Mag, Phase (degrees) ]:"; Ts "Sample time:"
      mask help:
      | Power Factor Block developed by Dr Rodney Tan
      | Version 1.01 (Aug 2016)
      |
      | Compute power factor and phase angle of AC circuit voltage-current pair at fundamental frequency.
      |
      | The computation is based on Power block and Complex number function block.
      |
      | For the first cycle of simulation, the outputs are held constant to the powers computed for the Voltage initial input and Current initial input parameters.
      mask Help:
      | <b>Fundamental Frequency (Hz)</b>
      | Specify the measurement fundamental frequency, in hertz, of the input signal.
      | 
      | <b>Voltage initial input [ Mag, Phase (degrees) ]</b>
      | Specify the voltage initial magnitude and phase to set a constant output for the first cycle of simulation.
      | 
      | <b>Current initial input [ Mag, Phase (degrees) ]</b>
      | Specify the current initial magnitude and phase to set a constant output for the first cycle of simulation.
      | 
      | <b>Sample Time</b>
      | Specify the sample time of the block, in seconds. Set to 0 to implement a continuous block.
      mask TypeOptions Freq: Power/Freq
      mask TypeOptions Vinit: Power/Vinit
      mask TypeOptions Iinit: Power/Iinit
      mask TypeOptions Ts: Power/Ts
  Power Factor1 : Display
  Scope : Scope  Commented=on
  THD : spsTHDLib/THD  Freq=60  Ts=Ts_Power
  THD (% and signal) : Scope  NumInputPorts=2
  THD (%) : Display
      settings: Format=bank
  THD1 : spsTHDLib/THD  Freq=60  Ts=Ts_Power
  Vabc pu1 : Scope
  to % : Gain  Gain=100  SampleTime=Ts_Power
  to %1 : Gain  Gain=100  SampleTime=Ts_Power
  ángulo de V (%)1 : Display  Commented=on
      settings: Format=bank
  tag scope: PFabc_Bus4=global, THDi_abc_Bus4=global, THDv_abc_Bus4=global
  wires:
  [IabcLL_Bus_4] -> THD1/1, Power Factor Block1/2(Iabc)
  THD/1 -> to %/1
  Power Factor Block1/4(Iabc y Iabc (rms)) -> Measurement1/4
  Power Factor Block1/1(Pabc) -> Measurement1/1
  Conv pu1/1 -> Vabc pu1/1
  Power Factor Block1/2(Qabc) -> Measurement1/2
  Power Factor Block1/3(Vabc y Vabc (rms)) -> Conv pu1/1, Measurement1/3
  Power Factor Block1/5("PFabc ") -> [PFabc_Bus4], Power Factor1/1
  to %/1 -> [THDv_abc_Bus4], THD (%)/1, THD (% and signal)/2  "THD (%)"
  Conv pu2/1 -> PLL/1(Vabc_LN_pu)
  PLL/1(delta_abc) -> Current2/1, Scope/1, ángulo de V (%)1/1
  [VabcLL_Bus_4] -> Power Factor Block1/1(Vabc), Conv pu2/1, THD/1, THD (% and signal)/1  "Signal Vabc"
  THD1/1 -> to %1/1
  to %1/1 -> [THDi_abc_Bus4]  "THD (%)"

== system Model_14Bus_Microgrid_paper_Latam/Bus_6  ==
  note: C
  note: B
  note: A
  note: C
  note: Linea - Neutro
  note: B
  note: A
  note: A
  note: B
  Conv pu1 : Gain  Gain=sqrt (3) /Vnom_prim  SaturateOnIntegerOverflow=on  OutDataTypeStr=Inherit: Same as input  ParamDataTypeStr=Inherit: Same as input
  Conv pu2 : Gain  Commented=on  Gain=sqrt (3) /Vnom_prim  SaturateOnIntegerOverflow=on  OutDataTypeStr=Inherit: Same as input  ParamDataTypeStr=Inherit: Same as input
  Current2 : Goto  Commented=on  GotoTag=delta_abc_Bus6  TagVisibility=global
  Measurement1 : Scope  NumInputPorts=4
  PLL : Subsystem  Commented=on
  PLL (3ph) : spsPLL3phLib/PLL (3ph)  Commented=on  Fmin=45  Par_Init=[0, 60]  ParK=[180, 3200, 1]  TcD=1e-4  MaxRateChangeFreq=12  FilterCutOffFreq=25  Ts=0  AGC=on
  Power Factor Block1 : Subsystem  mask(Power Factor Block){Freq=Fnom, Vinit=[0, 0], Iinit=[0, 0], Ts=0}
      mask prompts: Freq "Fundamental frequency (Hz):"; Vinit "Voltage initial input [ Mag, Phase (degrees) ]:"; Iinit "Current initial input [ Mag, Phase (degrees) ]:"; Ts "Sample time:"
      mask help:
      | Power Factor Block developed by Dr Rodney Tan
      | Version 1.01 (Aug 2016)
      |
      | Compute power factor and phase angle of AC circuit voltage-current pair at fundamental frequency.
      |
      | The computation is based on Power block and Complex number function block.
      |
      | For the first cycle of simulation, the outputs are held constant to the powers computed for the Voltage initial input and Current initial input parameters.
      mask Help:
      | <b>Fundamental Frequency (Hz)</b>
      | Specify the measurement fundamental frequency, in hertz, of the input signal.
      | 
      | <b>Voltage initial input [ Mag, Phase (degrees) ]</b>
      | Specify the voltage initial magnitude and phase to set a constant output for the first cycle of simulation.
      | 
      | <b>Current initial input [ Mag, Phase (degrees) ]</b>
      | Specify the current initial magnitude and phase to set a constant output for the first cycle of simulation.
      | 
      | <b>Sample Time</b>
      | Specify the sample time of the block, in seconds. Set to 0 to implement a continuous block.
      mask TypeOptions Freq: Power/Freq
      mask TypeOptions Vinit: Power/Vinit
      mask TypeOptions Iinit: Power/Iinit
      mask TypeOptions Ts: Power/Ts
  Power Factor1 : Display
  Scope : Scope  Commented=on
  Scope2 : Scope  Commented=on
  THD : spsTHDLib/THD  Freq=60  Ts=Ts_Power
  THD (% and signal) : Scope  NumInputPorts=2
  THD (%) : Display
      settings: Format=bank
  THD1 : spsTHDLib/THD  Freq=60  Ts=Ts_Power
  Terminator : Terminator  Commented=on
  Vabc pu1 : Scope
  frecuency (Hz) : Display  Commented=on
  to % : Gain  Gain=100  SampleTime=Ts_Power
  to %1 : Gain  Gain=100  SampleTime=Ts_Power
  ángulo de V (%)1 : Display  Commented=on
      settings: Format=bank
  tag scope: PFabc_Bus6=global, THDi_abc_Bus6=global, THDv_abc_Bus6=global
  wires:
  [IabcLL_Bus_6] -> THD1/1, Power Factor Block1/2(Iabc)
  THD/1 -> to %/1
  Power Factor Block1/4(Iabc y Iabc (rms)) -> Measurement1/4
  Power Factor Block1/1(Pabc) -> Measurement1/1
  Conv pu1/1 -> Vabc pu1/1
  Power Factor Block1/2(Qabc) -> Measurement1/2
  Power Factor Block1/3(Vabc y Vabc (rms)) -> Conv pu1/1, Measurement1/3
  Power Factor Block1/5("PFabc ") -> [PFabc_Bus6], Power Factor1/1
  to %/1 -> [THDv_abc_Bus6], THD (%)/1, THD (% and signal)/2  "THD (%)"
  PLL/1(delta_abc) -> Current2/1, Scope/1, ángulo de V (%)1/1
  Conv pu2/1 -> PLL/1(Vabc_LN_pu)
  PLL (3ph)/2 -> Terminator/1
  [VabcLL_Bus_6] -> Power Factor Block1/1(Vabc), Conv pu2/1, PLL (3ph)/1, THD/1, THD (% and signal)/1  "Vabc"
  PLL (3ph)/1 -> Scope2/1, frecuency (Hz)/1
  THD1/1 -> to %1/1
  to %1/1 -> [THDi_abc_Bus6]  "THD (%)"

== system Model_14Bus_Microgrid_paper_Latam/Bus_7 ==
  note: C
  note: B
  note: A
  note: C
  note: Linea - Neutro
  note: B
  note: A
  note: A
  note: B
  Conv pu1 : Gain  Gain=sqrt (3) /Vnom_prim  SaturateOnIntegerOverflow=on  OutDataTypeStr=Inherit: Same as input  ParamDataTypeStr=Inherit: Same as input
  Conv pu2 : Gain  Commented=on  Gain=sqrt (3) /Vnom_prim  SaturateOnIntegerOverflow=on  OutDataTypeStr=Inherit: Same as input  ParamDataTypeStr=Inherit: Same as input
  Current2 : Goto  Commented=on  GotoTag=delta_abc_Bus7  TagVisibility=global
  Measurement1 : Scope  NumInputPorts=4
  PLL : Subsystem  Commented=on
  PLL (3ph) : spsPLL3phLib/PLL (3ph)  Commented=on  Fmin=45  Par_Init=[0, 60]  ParK=[180, 3200, 1]  TcD=1e-4  MaxRateChangeFreq=12  FilterCutOffFreq=25  Ts=0  AGC=on
  Power Factor Block1 : Subsystem  mask(Power Factor Block){Freq=Fnom, Vinit=[0, 0], Iinit=[0, 0], Ts=0}
      mask prompts: Freq "Fundamental frequency (Hz):"; Vinit "Voltage initial input [ Mag, Phase (degrees) ]:"; Iinit "Current initial input [ Mag, Phase (degrees) ]:"; Ts "Sample time:"
      mask help:
      | Power Factor Block developed by Dr Rodney Tan
      | Version 1.01 (Aug 2016)
      |
      | Compute power factor and phase angle of AC circuit voltage-current pair at fundamental frequency.
      |
      | The computation is based on Power block and Complex number function block.
      |
      | For the first cycle of simulation, the outputs are held constant to the powers computed for the Voltage initial input and Current initial input parameters.
      mask Help:
      | <b>Fundamental Frequency (Hz)</b>
      | Specify the measurement fundamental frequency, in hertz, of the input signal.
      | 
      | <b>Voltage initial input [ Mag, Phase (degrees) ]</b>
      | Specify the voltage initial magnitude and phase to set a constant output for the first cycle of simulation.
      | 
      | <b>Current initial input [ Mag, Phase (degrees) ]</b>
      | Specify the current initial magnitude and phase to set a constant output for the first cycle of simulation.
      | 
      | <b>Sample Time</b>
      | Specify the sample time of the block, in seconds. Set to 0 to implement a continuous block.
      mask TypeOptions Freq: Power/Freq
      mask TypeOptions Vinit: Power/Vinit
      mask TypeOptions Iinit: Power/Iinit
      mask TypeOptions Ts: Power/Ts
  Power Factor1 : Display
  Scope : Scope  Commented=on
  Scope2 : Scope  Commented=on
  THD : spsTHDLib/THD  Freq=60  Ts=Ts_Power
  THD (% and signal) : Scope  NumInputPorts=2
  THD (%) : Display
      settings: Format=bank
  THD1 : spsTHDLib/THD  Freq=60  Ts=Ts_Power
  Terminator : Terminator  Commented=on
  Vabc pu1 : Scope
  frecuency (Hz) : Display  Commented=on
  to % : Gain  Gain=100  SampleTime=Ts_Power
  to %1 : Gain  Gain=100  SampleTime=Ts_Power
  ángulo de V (%)1 : Display  Commented=on
      settings: Format=bank
  tag scope: PFabc_Bus7=global, THDi_abc_Bus7=global, THDv_abc_Bus7=global
  wires:
  [IabcLL_Bus_7] -> THD1/1, Power Factor Block1/2(Iabc)
  THD/1 -> to %/1
  Power Factor Block1/4(Iabc y Iabc (rms)) -> Measurement1/4
  Power Factor Block1/1(Pabc) -> Measurement1/1
  Conv pu1/1 -> Vabc pu1/1
  Power Factor Block1/2(Qabc) -> Measurement1/2
  Power Factor Block1/3(Vabc y Vabc (rms)) -> Conv pu1/1, Measurement1/3
  to %/1 -> [THDv_abc_Bus7], THD (%)/1, THD (% and signal)/2  "THD (%)"
  Power Factor Block1/5("PFabc ") -> [PFabc_Bus7], Power Factor1/1
  PLL/1(delta_abc) -> Current2/1, Scope/1, ángulo de V (%)1/1
  Conv pu2/1 -> PLL/1(Vabc_LN_pu)
  [VabcLL_Bus_7] -> PLL (3ph)/1, Conv pu2/1, THD/1, THD (% and signal)/1, Power Factor Block1/1(Vabc)  "Vabc"
  PLL (3ph)/2 -> Terminator/1
  PLL (3ph)/1 -> Scope2/1, frecuency (Hz)/1
  THD1/1 -> to %1/1
  to %1/1 -> [THDi_abc_Bus7]  "THD (%)"

== system Model_14Bus_Microgrid_paper_Latam/Bus_9 ==
  note: C
  note: B
  note: A
  note: C
  note: Linea - Neutro
  note: B
  note: A
  note: A
  note: B
  Conv pu1 : Gain  Gain=sqrt (3) /Vnom_prim  SaturateOnIntegerOverflow=on  OutDataTypeStr=Inherit: Same as input  ParamDataTypeStr=Inherit: Same as input
  Conv pu2 : Gain  Commented=on  Gain=sqrt (3) /Vnom_prim  SaturateOnIntegerOverflow=on  OutDataTypeStr=Inherit: Same as input  ParamDataTypeStr=Inherit: Same as input
  Current2 : Goto  Commented=on  GotoTag=delta_abc_Bus9  TagVisibility=global
  Measurement1 : Scope  NumInputPorts=4
  PLL : Subsystem  Commented=on
  Power Factor Block1 : Subsystem  mask(Power Factor Block){Freq=Fnom, Vinit=[0, 0], Iinit=[0, 0], Ts=0}
      mask prompts: Freq "Fundamental frequency (Hz):"; Vinit "Voltage initial input [ Mag, Phase (degrees) ]:"; Iinit "Current initial input [ Mag, Phase (degrees) ]:"; Ts "Sample time:"
      mask help:
      | Power Factor Block developed by Dr Rodney Tan
      | Version 1.01 (Aug 2016)
      |
      | Compute power factor and phase angle of AC circuit voltage-current pair at fundamental frequency.
      |
      | The computation is based on Power block and Complex number function block.
      |
      | For the first cycle of simulation, the outputs are held constant to the powers computed for the Voltage initial input and Current initial input parameters.
      mask Help:
      | <b>Fundamental Frequency (Hz)</b>
      | Specify the measurement fundamental frequency, in hertz, of the input signal.
      | 
      | <b>Voltage initial input [ Mag, Phase (degrees) ]</b>
      | Specify the voltage initial magnitude and phase to set a constant output for the first cycle of simulation.
      | 
      | <b>Current initial input [ Mag, Phase (degrees) ]</b>
      | Specify the current initial magnitude and phase to set a constant output for the first cycle of simulation.
      | 
      | <b>Sample Time</b>
      | Specify the sample time of the block, in seconds. Set to 0 to implement a continuous block.
      mask TypeOptions Freq: Power/Freq
      mask TypeOptions Vinit: Power/Vinit
      mask TypeOptions Iinit: Power/Iinit
      mask TypeOptions Ts: Power/Ts
  Power Factor1 : Display
  Scope : Scope  Commented=on
  THD : spsTHDLib/THD  Freq=60  Ts=Ts_Power
  THD (% and signal) : Scope  NumInputPorts=2
  THD (%) : Display
      settings: Format=bank
  THD1 : spsTHDLib/THD  Freq=60  Ts=Ts_Power
  Vabc pu1 : Scope
  to % : Gain  Gain=100  SampleTime=Ts_Power
  to %1 : Gain  Gain=100  SampleTime=Ts_Power
  ángulo de V (%)1 : Display  Commented=on
      settings: Format=bank
  tag scope: PFabc_Bus9=global, THDi_abc_Bus9=global, THDv_abc_Bus9=global
  wires:
  [IabcLL_Bus_9] -> THD1/1, Power Factor Block1/2(Iabc)
  THD/1 -> to %/1
  Power Factor Block1/4(Iabc y Iabc (rms)) -> Measurement1/4
  Power Factor Block1/1(Pabc) -> Measurement1/1
  Conv pu1/1 -> Vabc pu1/1
  Power Factor Block1/2(Qabc) -> Measurement1/2
  Power Factor Block1/3(Vabc y Vabc (rms)) -> Conv pu1/1, Measurement1/3
  to %/1 -> [THDv_abc_Bus9], THD (%)/1, THD (% and signal)/2  "THD (%)"
  Power Factor Block1/5("PFabc ") -> [PFabc_Bus9], Power Factor1/1
  PLL/1(delta_abc) -> Current2/1, Scope/1, ángulo de V (%)1/1
  [VabcLL_Bus_9] -> Conv pu2/1, THD/1, THD (% and signal)/1, Power Factor Block1/1(Vabc)  "Signal Vabc"
  Conv pu2/1 -> PLL/1(Vabc_LN_pu)
  THD1/1 -> to %1/1
  to %1/1 -> [THDi_abc_Bus9]  "THD (%)"

== system Model_14Bus_Microgrid_paper_Latam/Bus_slack  ==
  note: C
  note: B
  note: A
  note: C
  note: Linea - Neutro
  note: B
  note: A
  note: A
  note: B
  note: C
  Conv pu1 : Gain  Gain=sqrt (3) /Vnom_prim  SaturateOnIntegerOverflow=on  OutDataTypeStr=Inherit: Same as input  ParamDataTypeStr=Inherit: Same as input
  Conv pu2 : Gain  Gain=sqrt (3) /Vnom_prim  SaturateOnIntegerOverflow=on  OutDataTypeStr=Inherit: Same as input  ParamDataTypeStr=Inherit: Same as input
  Measurement1 : Scope  NumInputPorts=4
  PLL : Subsystem
  PLL (3ph) : spsPLL3phLib/PLL (3ph)  Fmin=45  Par_Init=[0, 60]  ParK=[180, 3200, 1]  TcD=1e-4  MaxRateChangeFreq=12  FilterCutOffFreq=25  Ts=0  AGC=on
  Power Factor Block1 : Subsystem  mask(Power Factor Block){Freq=Fnom, Vinit=[0, 0], Iinit=[0, 0], Ts=0}
      mask prompts: Freq "Fundamental frequency (Hz):"; Vinit "Voltage initial input [ Mag, Phase (degrees) ]:"; Iinit "Current initial input [ Mag, Phase (degrees) ]:"; Ts "Sample time:"
      mask help:
      | Power Factor Block developed by Dr Rodney Tan
      | Version 1.01 (Aug 2016)
      |
      | Compute power factor and phase angle of AC circuit voltage-current pair at fundamental frequency.
      |
      | The computation is based on Power block and Complex number function block.
      |
      | For the first cycle of simulation, the outputs are held constant to the powers computed for the Voltage initial input and Current initial input parameters.
      mask Help:
      | <b>Fundamental Frequency (Hz)</b>
      | Specify the measurement fundamental frequency, in hertz, of the input signal.
      | 
      | <b>Voltage initial input [ Mag, Phase (degrees) ]</b>
      | Specify the voltage initial magnitude and phase to set a constant output for the first cycle of simulation.
      | 
      | <b>Current initial input [ Mag, Phase (degrees) ]</b>
      | Specify the current initial magnitude and phase to set a constant output for the first cycle of simulation.
      | 
      | <b>Sample Time</b>
      | Specify the sample time of the block, in seconds. Set to 0 to implement a continuous block.
      mask TypeOptions Freq: Power/Freq
      mask TypeOptions Vinit: Power/Vinit
      mask TypeOptions Iinit: Power/Iinit
      mask TypeOptions Ts: Power/Ts
  Power Factor1 : Display
  Scope : Scope
  Scope2 : Scope
  THD : spsTHDLib/THD  Freq=60  Ts=Ts_Power
  THD (% and signal) : Scope  NumInputPorts=2
  THD (%) : Display
      settings: Format=bank
  THD1 : spsTHDLib/THD  Freq=60  Ts=Ts_Power
  Terminator : Terminator
  Vabc pu1 : Scope
  frecuency (Hz) : Display
  to % : Gain  Gain=100  SampleTime=Ts_Power
  to %1 : Gain  Gain=100  SampleTime=Ts_Power
  ángulo de V (%)1 : Display
      settings: Format=bank
  tag scope: PFabc_Bus13=global, THDi_abc_Bus13=global, THDv_abc_Bus13=global, delta_abc_Bus13=global
  wires:
  [Iabc_Sec] -> THD1/1, Power Factor Block1/2(Iabc)  "Signal Iabc"
  THD/1 -> to %/1
  Power Factor Block1/4(Iabc y Iabc (rms)) -> Measurement1/4
  Power Factor Block1/1(Pabc) -> Measurement1/1
  Conv pu1/1 -> Vabc pu1/1
  Power Factor Block1/2(Qabc) -> Measurement1/2
  Power Factor Block1/3(Vabc y Vabc (rms)) -> Conv pu1/1, Measurement1/3
  to %/1 -> [THDv_abc_Bus13], THD (%)/1, THD (% and signal)/2  "THD (%)"
  Power Factor Block1/5("PFabc ") -> [PFabc_Bus13], Power Factor1/1
  Conv pu2/1 -> PLL/1(Vabc_LN_pu)
  PLL/1(delta_abc) -> [delta_abc_Bus13], Scope/1, ángulo de V (%)1/1
  [Vabc_Sec] -> Power Factor Block1/1(Vabc), THD/1, THD (% and signal)/1, PLL (3ph)/1, Conv pu2/1  "Vabc"
  PLL (3ph)/2 -> Terminator/1
  PLL (3ph)/1 -> Scope2/1, frecuency (Hz)/1
  THD1/1 -> to %1/1
  to %1/1 -> [THDi_abc_Bus13]  "THD (%)"

== system Model_14Bus_Microgrid_paper_Latam/Diesel_ 3MVA ==
  note: Diesel generator 2
  2.4kV  50MVA : spsThreePhaseSeriesRLCBranchLib/Three-Phase Series RLC Branch  LConnTagsString=A|B|C  RConnTagsString=A|B|C  BranchType=RL  Resistance=2.4e3^2/50e6/10  Inductance=2.4e3^2/50e6/(2*pi*60)  Capacitance=1.0  Measurements=None
  Ground1 : spsGroundLib/Ground  LConnTagsString=a
  Programmable Voltage Source1 : spsThreePhaseProgrammableVoltageSourceLib/Three-Phase Programmable Voltage Source  PositiveSequence="[Vnom_Diesel*0.9848 -60  Fnom]"  VariationEntity=None  VariationType=Table of time-amplitude pairs  VariationTypeAlt=Step  VariationStep=-0.3  VariationRate=0.5  VariationMagnitude=0.4  VariationFrequency=2  VariationTiming=[0.1 1.2]  VariationPhaseA=off  Amplitudes=[1]  TimeValues=[0]  HarmonicGeneration=off  HarmonicA=[3 0.2 -25 0]  HarmonicB="[2 0.15  35 2]"  Timing="[0.1  0.6]"  BusType=PV  Pref=Pgen_Diesel  Qref=0  Qmin=-inf  Qmax=inf
  a1 : PMIOPort  Tag=PMCPort  Side=Left
  b1 : PMIOPort  Tag=PMCPort  Port=2  Side=Left
  c1 : PMIOPort  Tag=PMCPort  Port=3  Side=Left
  connections:
  Programmable Voltage Source1/RConn3 -- 2.4kV  50MVA/LConn3
  Ground1/LConn1 -- Programmable Voltage Source1/LConn1
  Programmable Voltage Source1/RConn2 -- 2.4kV  50MVA/LConn2
  2.4kV  50MVA/LConn1 -- Programmable Voltage Source1/RConn1
  b1/RConn1 -- 2.4kV  50MVA/RConn2
  a1/RConn1 -- 2.4kV  50MVA/RConn1
  c1/RConn1 -- 2.4kV  50MVA/RConn3

== system Model_14Bus_Microgrid_paper_Latam/Line 1 (150m) ==
  Bus_14 3 : Subsystem  Commented=on
  Goto6 : Goto  Commented=on  GotoTag=Ia_L1  TagVisibility=global
  Goto7 : Goto  Commented=on  GotoTag=Ib_L1  TagVisibility=global
  Goto8 : Goto  Commented=on  GotoTag=Ic_L1  TagVisibility=global
  Ia_L1 : spsCurrentMeasurementLib/Current Measurement  PhasorSimulation=off  OutputType=Complex  PSBequivalent=0
  Ib_L1 : spsCurrentMeasurementLib/Current Measurement  PhasorSimulation=off  OutputType=Complex  PSBequivalent=0
  Ic_L1 : spsCurrentMeasurementLib/Current Measurement  PhasorSimulation=off  OutputType=Complex  PSBequivalent=0
  Line1 150m : spsThreePhaseSeriesRLCBranchLib/Three-Phase Series RLC Branch  LConnTagsString=A|B|C  RConnTagsString=A|B|C  BranchType=RL  Resistance=Rls * dis1  Inductance=Xls / 377 * dis1  Capacitance=1e-6  Measurements=None
  B : PMIOPort  Port=2  Side=Left
  A : PMIOPort  Side=Left
  C : PMIOPort  Port=3  Side=Left
  a : PMIOPort  Port=4  Side=Right
  b : PMIOPort  Port=5  Side=Right
  c : PMIOPort  Port=6  Side=Right
  wires:
  Ib_L1/1 -> Goto7/1
  Ia_L1/1 -> Goto6/1
  Ic_L1/1 -> Goto8/1
  connections:
  A/RConn1 -- Ia_L1/RConn1
  C/RConn1 -- Ic_L1/RConn1
  B/RConn1 -- Ib_L1/RConn1
  Line1 150m/RConn1 -- a/RConn1
  Line1 150m/LConn3 -- Ic_L1/LConn1
  Line1 150m/LConn2 -- Ib_L1/LConn1
  Line1 150m/LConn1 -- Ia_L1/LConn1
  Line1 150m/RConn2 -- b/RConn1
  Line1 150m/RConn3 -- c/RConn1
